simulink model "KUKA_KR10_R1100_1D"  (R2023b)
settings: Solver=ode15s  StartTime=0.0  StopTime=3  RelTol=1e-9  AbsTol=1e-9  EnableMultiTasking=on
values from neighbouring files (symbols this model uses):
  N = length(accelX)    [pds.m]
undefined symbols (not defined in the file or in its folder): X, Y, Z
libraries: nesl_utility x50, sm_lib x46
(part 1 of 2)
settings Model: Creator=beth0005  LastModifiedBy=Johannes
settings SolverCC: AutoScaleAbsTol=off  AlgebraicLoopSolver=TrustRegion
settings DataIOCC: LimitDataPoints=on  MaxDataPoints=10000
settings OptimizationCC: LifeSpan=inf
settings DebuggingCC: UnconnectedInputMsg=warning  UnconnectedOutputMsg=warning  UnconnectedLineMsg=warning  AllowSymbolicDim=off  SFUnexpectedBacktrackingDiag=warning  SFNoUnconditionalDefaultTransitionDiag=warning  SFExecutionAtInitializationDiag=none  ArithmeticOperatorsInVariantConditions=warning
settings ModelReferenceCC: EnableRefExpFcnMdlSchedulingChecks=on
settings SFSimCC: SimUseLocalCustomCode=off  CustomCodeUndefinedFunction=UseInterfaceOnly
settings RTWCC: RTWUseLocalCustomCode=off  DLArmComputeVersion=19.05
settings CodeAppCC: StateflowObjectComments=on
settings GRTTargetCC: TargetLangStandard=C89/C90 (ANSI)
settings ConfigComp: CovMetricSettings=dw  CovSaveCumulativeToWorkspaceVar=on  CovSaveSingleToWorkspaceVar=on  CovExternalEMLEnable=off  CovSFcnEnable=off
settings SimscapeCC: SimscapeLogType=all  SimscapeLogSimulationStatistics=on  SimscapeLogDataHistory=10000

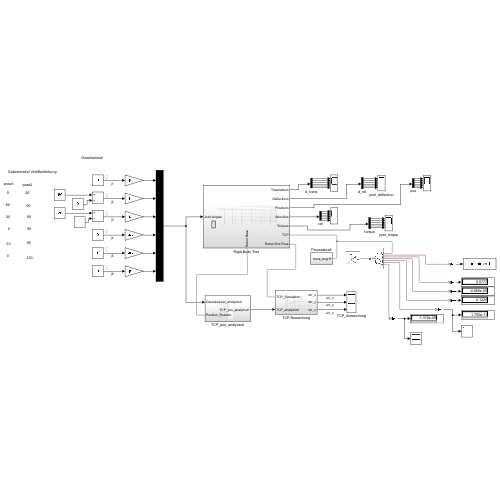
[thumbnail: Simulink's stored preview of the top-level diagram]
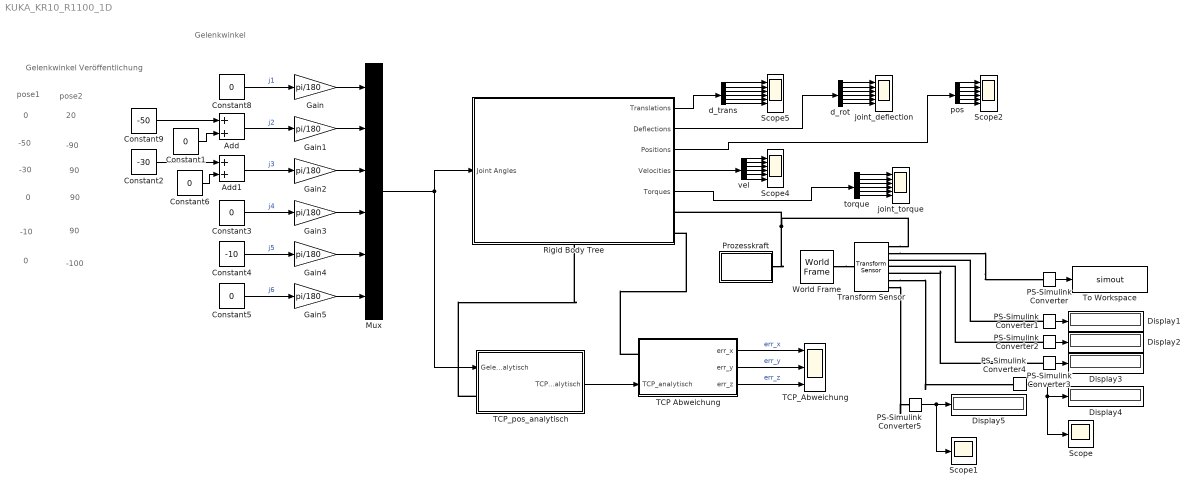
== system KUKA_KR10_R1100_1D ==
  note: -100
  note: pose2
  note: pose1
  note: 90
  note: 90
  note: 20
  note: 90
  note: -90
  note: Gelenkwinkel Veröffentlichung
  note: Gelenkwinkel
  note: 0
  note: -10
  note: 0
  note: 0
  note: -30
  note: -50
  Add : Sum
  Add1 : Sum
  Constant{1,3,5..6,8} (5 alike) : Constant  Value=0
  Constant2 : Constant  Value=-30
  Constant4 : Constant  Value=-10
  Constant9 : Constant  Value=-50
  Display{1..5} (5 alike) : Display
  Gain{,1..5} (6 alike) : Gain  Gain=pi/180
  Mux : Mux  Inputs=6
  PS-Simulink Converter{,1..5} (6 alike) : nesl_utility/PS-Simulink Converter  PhysicalDomain=network_engine_domain  SubClassName=ps_output  LeftPortType=input  RightPortType=output  PseudoPeriodic=off  Frequencies=[]  VectorFormat=inherit  Unit=inherit  AffineConversion=off
  Prozesskraft : Subsystem
  Rigid Body Tree : Subsystem
      settings: PortSchema="{\"entries\":[{\"content\":{\"sides\":[{\"content\":{\"connectorIds\":[\"In1\"]},\"type\":\"ConnectorPlacement.EquallySpacedRectSide\",\"uuid\":\"62483687-f9cb-4c30-88aa-fbca99035508\"},{\"content\":{\"connectorIds\":[\"Out1\",\"Out2\",\"Out3\",\"Out4\",\"Out5\",\"RConn1\",\"RConn2\"],\"side\":\"RIGHT\"},\"type\":\"ConnectorPlacement.EquallySpacedRectSide\",\"uuid\":\"72747b39-4529-4d6b-bc1f-f243ab09c1ee\"},{\"content\":{\"side\":\"TOP\"},\"type\":\"ConnectorPlacement.EquallySpacedRectSide\",\"uuid\":\"6a7c85b5-1fcd-47a7-a71b-25055be44f92\"},{\"content\":{\"connectorIds\":[\"RConn3\"],\"side\":\"BOTTOM\"},\"type\":\"ConnectorPlacement.EquallySpacedRectSide\",\"uuid\":\"78c07802-d245-487e-84d6-9da01077e918\"}]},\"type\":\"ConnectorPlacement.EquallySpacedConnector\",\"uuid\":\"7be79213-6e9f-4572-8e99-74e3fd1a1f63\"}],\"packageUris\":[\"http://schema.mathworks.com/mf0/Connector/R2020b\"],\"version\":\"1.0\"}"
  Scope : Scope
  Scope1 : Scope
  Scope2 : Scope  NumInputPorts=6
  Scope4 : Scope  NumInputPorts=6
  Scope5 : Scope  NumInputPorts=6
  TCP Abweichung : Subsystem
      settings: PortSchema="{\"entries\":[{\"content\":{\"sides\":[{\"content\":{\"connectorIds\":[\"LConn1\",\"In1\"]},\"type\":\"ConnectorPlacement.EquallySpacedRectSide\",\"uuid\":\"8fbb3f34-d7d1-4090-9281-a387436a6191\"},{\"content\":{\"connectorIds\":[\"Out1\",\"Out2\",\"Out3\"],\"side\":\"RIGHT\"},\"type\":\"ConnectorPlacement.EquallySpacedRectSide\",\"uuid\":\"2461bf91-e690-4063-84b2-ad7cc9454b37\"},{\"content\":{\"side\":\"TOP\"},\"type\":\"ConnectorPlacement.EquallySpacedRectSide\",\"uuid\":\"0fbb9cfb-49b2-42f2-b0a5-a9e967349aea\"}]},\"type\":\"ConnectorPlacement.EquallySpacedConnector\",\"uuid\":\"5e1e4f46-aaa2-4a76-a14e-db38171314b7\"}],\"packageUris\":[\"http://schema.mathworks.com/mf0/Connector/R2020b\"],\"version\":\"1.0\"}"
  TCP_Abweichung : Scope  NumInputPorts=3
  TCP_pos_analytisch : Subsystem
  To Workspace : ToWorkspace  VariableName=simout  SaveFormat=Structure  SampleTime=-1
  Transform Sensor : sm_lib/Frames and Transforms/Transform Sensor  MeasurementFrame=World  RotationSequence=XYX  SenseAngle=off  SenseAxis=off  SenseQ=off  SenseR=on  SenseRotationSequence=off  SenseOmegaX=off  SenseOmegaY=off  SenseOmegaZ=off  SenseOmega=off  SenseQDot=off  SenseRDot=off  SenseRotationSequenceDot=off  SenseAlphaX=off  SenseAlphaY=off  SenseAlphaZ=off  SenseAlpha=off  SenseQDDot=off  SenseRDDot=off  SenseX=on  SenseY=on  SenseZ=on  SenseXYZ=off  SenseRad=off  SenseAzim=off  SenseDist=off  SenseInc=off  SenseXDot=off  SenseYDot=off  SenseZDot=off  SenseXYZDot=on  SenseRadDot=off  SenseAzimDot=off  SenseDistDot=off  SenseIncDot=off  SenseXDDot=off  SenseYDDot=off  SenseZDDot=off  SenseXYZDDot=on  SenseRadDDot=off  SenseAzimDDot=off  SenseDistDDot=off  SenseIncDDot=off
  World Frame : sm_lib/Frames and Transforms/World Frame
  d_rot : Demux  Outputs=6
  d_trans : Demux  Outputs=6
  joint_deflection : Scope  NumInputPorts=6
  joint_torque : Scope  NumInputPorts=6
  pos : Demux  Outputs=6
  torque : Demux  Outputs=6
  vel : Demux  Outputs=6
  wires:
  Constant5/1 -> Gain5/1  "j6"
  Constant4/1 -> Gain4/1  "j5"
  Constant3/1 -> Gain3/1  "j4"
  d_rot/3 -> joint_deflection/3
  d_rot/6 -> joint_deflection/6
  d_rot/4 -> joint_deflection/4
  d_rot/5 -> joint_deflection/5
  d_rot/2 -> joint_deflection/2
  d_rot/1 -> joint_deflection/1
  pos/1 -> Scope2/1
  pos/2 -> Scope2/2
  pos/5 -> Scope2/5
  pos/4 -> Scope2/4
  pos/6 -> Scope2/6
  pos/3 -> Scope2/3
  torque/3 -> joint_torque/3
  torque/6 -> joint_torque/6
  torque/4 -> joint_torque/4
  torque/5 -> joint_torque/5
  torque/2 -> joint_torque/2
  torque/1 -> joint_torque/1
  vel/1 -> Scope4/1
  vel/2 -> Scope4/2
  vel/5 -> Scope4/5
  vel/4 -> Scope4/4
  vel/6 -> Scope4/6
  vel/3 -> Scope4/3
  d_trans/1 -> Scope5/1
  d_trans/2 -> Scope5/2
  d_trans/5 -> Scope5/5
  d_trans/4 -> Scope5/4
  d_trans/6 -> Scope5/6
  d_trans/3 -> Scope5/3
  TCP_pos_analytisch/1(TCP_pos_analytisch) -> TCP Abweichung/1(TCP_analytisch)
  TCP Abweichung/1(err_x) -> TCP_Abweichung/1  "err_x"
  TCP Abweichung/2(err_y) -> TCP_Abweichung/2  "err_y"
  TCP Abweichung/3(err_z) -> TCP_Abweichung/3  "err_z"
  Constant8/1 -> Gain/1  "j1"
  Gain/1 -> Mux/1
  Gain1/1 -> Mux/2
  Add/1 -> Gain1/1  "j2"
  Gain2/1 -> Mux/3
  Gain3/1 -> Mux/4
  Gain4/1 -> Mux/5
  Gain5/1 -> Mux/6
  Constant1/1 -> Add/2
  Constant6/1 -> Add1/2
  Add1/1 -> Gain2/1  "j3"
  PS-Simulink Converter1/1 -> Display1/1
  PS-Simulink Converter2/1 -> Display2/1
  PS-Simulink Converter3/1 -> Display3/1
  PS-Simulink Converter/1 -> To Workspace/1
  Constant9/1 -> Add/1
  Constant2/1 -> Add1/1
  PS-Simulink Converter4/1 -> Scope/1, Display4/1
  PS-Simulink Converter5/1 -> Scope1/1, Display5/1
  Mux/1 -> TCP_pos_analytisch/1(Gelenkwinkel_analytisch), Rigid Body Tree/1(Joint Angles)
  Rigid Body Tree/1(Translations) -> d_trans/1
  Rigid Body Tree/2(Deflections) -> d_rot/1
  Rigid Body Tree/3(Positions) -> pos/1
  Rigid Body Tree/4(Velocities) -> vel/1
  Rigid Body Tree/5(Torques) -> torque/1
  connections:
  World Frame/RConn1 -- Transform Sensor/LConn1
  Transform Sensor/RConn2 -- PS-Simulink Converter/LConn1
  PS-Simulink Converter1/LConn1 -- Transform Sensor/RConn3
  PS-Simulink Converter2/LConn1 -- Transform Sensor/RConn4
  PS-Simulink Converter3/LConn1 -- Transform Sensor/RConn5
  Transform Sensor/RConn6 -- PS-Simulink Converter4/LConn1
  Transform Sensor/RConn7 -- PS-Simulink Converter5/LConn1
  Prozesskraft/LConn1 -- Rigid Body Tree/RConn1 -- Transform Sensor/RConn1
  TCP_pos_analytisch/LConn1 -- Rigid Body Tree/RConn3
  TCP Abweichung/LConn1 -- Rigid Body Tree/RConn2

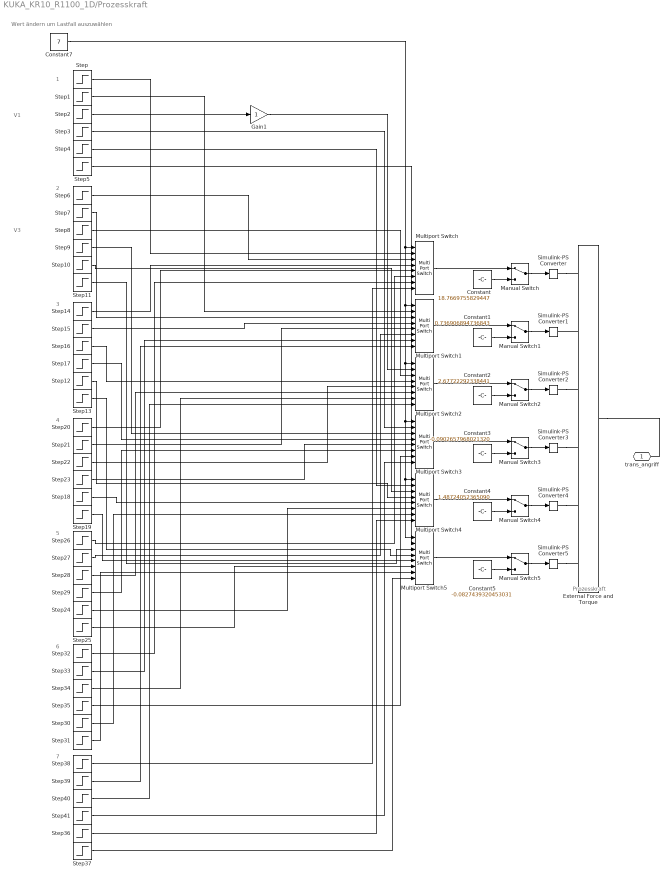
== system KUKA_KR10_R1100_1D/Prozesskraft ==
  note: Wert ändern um Lastfall auszuwählen
  note: V3
  note: V1
  note: Prozesskraft
  note: 1
  note: 2
  note: 3
  note: 4
  note: 5
  note: 6
  note: 7
  Constant : Constant  Value=18.7669755829447
  Constant1 : Constant  Value=0.736906894736843
  Constant2 : Constant  Value=2.67722292338441
  Constant3 : Constant  Value=-0.0902657968021320
  Constant4 : Constant  Value=1.48724052365090
  Constant5 : Constant  Value=-0.0827439320453031
  Constant7 : Constant  Value=7
  External Force and Torque : sm_lib/Forces and Torques/External Force and Torque  ForceResolutionFrame=AttachedFrame  EnableForceX=on  EnableForceY=on  EnableForceZ=on  EnableForce=off  TorqueResolutionFrame=AttachedFrame  EnableTorqueX=on  EnableTorqueY=on  EnableTorqueZ=on  EnableTorque=off
  Gain1 : Gain
  Manual Switch{,1..5} (6 alike) : ManualSwitch
  Multiport Switch{,1..5} (6 alike) : MultiPortSwitch  Inputs=7  SaturateOnIntegerOverflow=off  InputSameDT=off
  Simulink-PS Converter{,1..5} (6 alike) : nesl_utility/Simulink-PS Converter  PhysicalDomain=network_engine_domain  SubClassName=ps_input  LeftPortType=input  RightPortType=output  PseudoPeriodic=off  Frequencies=[]  NoiseDistribution=none  NoiseParameters=[]  Unit=1  AffineConversion=off  FilteringAndDerivatives=filter  SimscapeFilterOrder=2  InputFilterTimeConstant=0.001  UdotUserProvided=0
  Step : Step  Time=1.5  Before=10.45  After=0  SampleTime=0
  Step1 : Step  Time=1.5  Before=42.37  After=0  SampleTime=0
  Step10 : Step  Time=1.5  Before=0.27  After=0  SampleTime=0
  Step11 : Step  Time=1.5  Before=1.38  After=1.74  SampleTime=0
  Step12 : Step  Time=1.5  Before=0.47  After=0  SampleTime=0
  Step13 : Step  Time=1.5  Before=2.07  After=2.64  SampleTime=0
  Step14 : Step  Time=1.5  Before=8.44  After=0  SampleTime=0
  Step15 : Step  Time=1.5  Before=60.03  After=0  SampleTime=0
  Step16 : Step  Time=1.5  Before=-13.44  After=-47.67  SampleTime=0
  Step17 : Step  Time=1.5  Before=-0.03  After=0  SampleTime=0
  Step18 : Step  Time=1.5  Before=0.16  After=0  SampleTime=0
  Step19 : Step  Time=1.5  Before=2.36  After=3.01  SampleTime=0
  Step2 : Step  Time=1.5  Before=-7.82  After=-23.46  SampleTime=0
  Step20 : Step  Time=1.5  Before=6.32  After=0  SampleTime=0
  Step21 : Step  Time=1.5  Before=67.65  After=0  SampleTime=0
  Step22 : Step  Time=1.5  Before=-4.46  After=-25.52  SampleTime=0
  Step23 : Step  Time=1.5  Before=-0.02  After=0  SampleTime=0
  Step24 : Step  Time=1.5  Before=0.32  After=0  SampleTime=0
  Step25 : Step  Time=1.5  Before=3.54  After=4.54  SampleTime=0
  Step26 : Step  Time=1.5  Before=2.19  After=0  SampleTime=0
  Step27 : Step  Time=1.5  Before=102.5  After=0  SampleTime=0
  Step28 : Step  Time=1.5  Before=-9.11  After=-44.25  SampleTime=0
  Step29 : Step  Time=1.5  Before=-0.04  After=0  SampleTime=0
  Step3 : Step  Time=1.5  After=0  SampleTime=0
  Step30 : Step  Time=1.5  Before=0.3  After=0  SampleTime=0
  Step31 : Step  Time=1.5  Before=3.21  After=4.14  SampleTime=0
  Step32 : Step  Time=1.5  Before=1.98  After=0  SampleTime=0
  Step33 : Step  Time=1.5  Before=92.63  After=0  SampleTime=0
  Step34 : Step  Time=1.5  Before=-0.75  After=-22.78  SampleTime=0
  Step35 : Step  Time=1.5  Before=-0.03  After=0  SampleTime=0
  Step36 : Step  Time=1.5  Before=0.14  After=0  SampleTime=0
  Step37 : Step  Time=1.5  Before=4.83  After=6.22  SampleTime=0
  Step38 : Step  Time=1.5  Before=-5.57  After=0  SampleTime=0
  Step39 : Step  Time=1.5  Before=139.8  After=0  SampleTime=0
  Step4 : Step  Time=1.5  After=0  SampleTime=0
  Step40 : Step  Time=1.5  Before=-4.21  After=-40.32  SampleTime=0
  Step41 : Step  Time=1.5  Before=-0.05  After=0  SampleTime=0
  Step5 : Step  Time=1.5  Before=-1.462  After=-1.462  SampleTime=0
  Step6 : Step  Time=1.5  Before=9.11  After=0  SampleTime=0
  Step7 : Step  Time=1.5  Before=39.76  After=0  SampleTime=0
  Step8 : Step  Time=1.5  Before=-7.59  After=-28.04  SampleTime=0
  Step9 : Step  Time=1.5  Before=-0.02  After=0  SampleTime=0
  trans_angriff : PMIOPort  Side=Left
  wires:
  Constant7/1 -> Multiport Switch5/1, Multiport Switch4/1, Multiport Switch3/1, Multiport Switch2/1, Multiport Switch1/1, Multiport Switch/1
  Step/1 -> Multiport Switch/2
  Step1/1 -> Multiport Switch1/2
  Step2/1 -> Gain1/1
  Step3/1 -> Multiport Switch3/2
  Step4/1 -> Multiport Switch4/2
  Step5/1 -> Multiport Switch5/2
  Step6/1 -> Multiport Switch/3
  Step7/1 -> Multiport Switch1/3
  Step8/1 -> Multiport Switch2/3
  Step9/1 -> Multiport Switch3/3
  Step10/1 -> Multiport Switch4/3
  Step11/1 -> Multiport Switch5/3
  Step14/1 -> Multiport Switch/4
  Step15/1 -> Multiport Switch1/4
  Step16/1 -> Multiport Switch2/4
  Step17/1 -> Multiport Switch3/4
  Step12/1 -> Multiport Switch4/4
  Step13/1 -> Multiport Switch5/4
  Step20/1 -> Multiport Switch/5
  Step21/1 -> Multiport Switch1/5
  Step22/1 -> Multiport Switch2/5
  Step23/1 -> Multiport Switch3/5
  Step18/1 -> Multiport Switch4/5
  Step19/1 -> Multiport Switch5/5
  Step26/1 -> Multiport Switch/6
  Step27/1 -> Multiport Switch1/6
  Step28/1 -> Multiport Switch2/6
  Step29/1 -> Multiport Switch3/6
  Step24/1 -> Multiport Switch4/6
  Step25/1 -> Multiport Switch5/6
  Step32/1 -> Multiport Switch/7
  Step33/1 -> Multiport Switch1/7
  Step34/1 -> Multiport Switch2/7
  Step35/1 -> Multiport Switch3/7
  Step30/1 -> Multiport Switch4/7
  Step31/1 -> Multiport Switch5/7
  Step38/1 -> Multiport Switch/8
  Step39/1 -> Multiport Switch1/8
  Step40/1 -> Multiport Switch2/8
  Step41/1 -> Multiport Switch3/8
  Step36/1 -> Multiport Switch4/8
  Step37/1 -> Multiport Switch5/8
  Gain1/1 -> Multiport Switch2/2
  Multiport Switch/1 -> Manual Switch/1
  Manual Switch/1 -> Simulink-PS Converter/1
  Multiport Switch1/1 -> Manual Switch1/1
  Multiport Switch2/1 -> Manual Switch2/1
  Manual Switch2/1 -> Simulink-PS Converter2/1
  Manual Switch3/1 -> Simulink-PS Converter3/1
  Manual Switch4/1 -> Simulink-PS Converter4/1
  Manual Switch5/1 -> Simulink-PS Converter5/1
  Multiport Switch3/1 -> Manual Switch3/1
  Multiport Switch4/1 -> Manual Switch4/1
  Multiport Switch5/1 -> Manual Switch5/1
  Constant/1 -> Manual Switch/2
  Constant1/1 -> Manual Switch1/2
  Constant2/1 -> Manual Switch2/2
  Constant3/1 -> Manual Switch3/2
  Constant4/1 -> Manual Switch4/2
  Constant5/1 -> Manual Switch5/2
  Manual Switch1/1 -> Simulink-PS Converter1/1
  connections:
  Simulink-PS Converter4/RConn1 -- External Force and Torque/LConn5
  Simulink-PS Converter5/RConn1 -- External Force and Torque/LConn6
  Simulink-PS Converter3/RConn1 -- External Force and Torque/LConn4
  External Force and Torque/LConn2 -- Simulink-PS Converter1/RConn1
  Simulink-PS Converter2/RConn1 -- External Force and Torque/LConn3
  Simulink-PS Converter/RConn1 -- External Force and Torque/LConn1
  External Force and Torque/RConn1 -- trans_angriff/RConn1

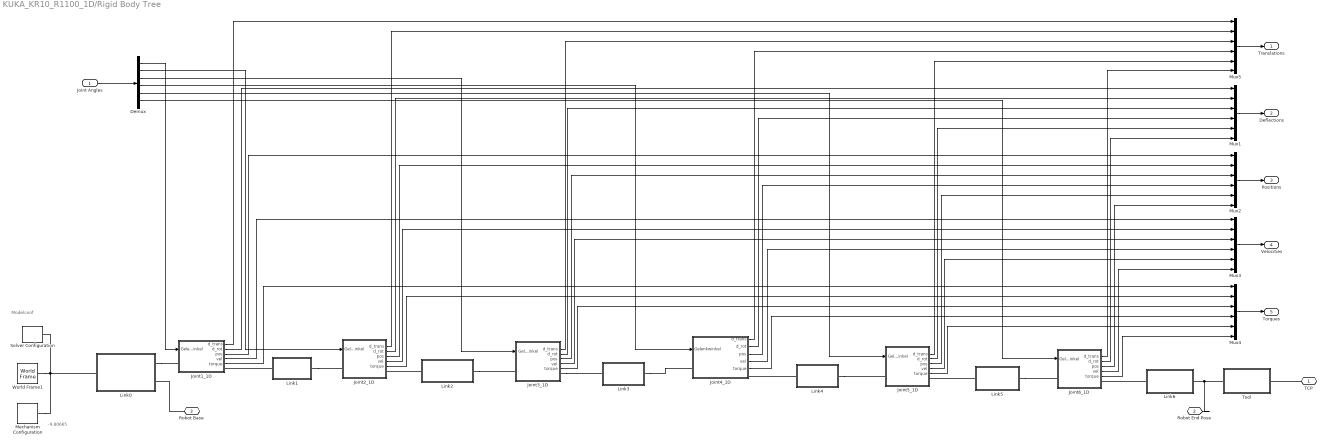
== system KUKA_KR10_R1100_1D/Rigid Body Tree ==
  note: Modelconf
  note: -9.80665
  Joint Angles : Inport
  Demux : Demux  Outputs=6
  Joint1_1D : Subsystem
  Joint2_1D : Subsystem
  Joint3_1D : Subsystem
  Joint4_1D : Subsystem
  Joint5_1D : Subsystem
  Joint6_1D : Subsystem
  Link0 : Subsystem
  Link1 : Subsystem
  Link2 : Subsystem
  Link3 : Subsystem
  Link4 : Subsystem
  Link5 : Subsystem
  Link6 : Subsystem
  Mechanism Configuration : sm_lib/Utilities/Mechanism Configuration  UniformGravity=Constant  GravityVector=[0 0 -9.80665]  GravityVectorUnits=m/s^2  LinearizationDelta=0.001  JointModeTransitionNonlinearIterations=2
  Mux{1..5} (5 alike) : Mux  Inputs=6
  Solver Configuration : nesl_utility/Solver Configuration  PhysicalDomain=network_engine_domain  SubClassName=solver  LeftPortType=input  RightPortType=generic  Tones=[]  Harmonics=[]  SimulateNoise=off  Profile=off  UseLocalSampling=off  EnableSwitchedLinearOptims=on  FrequencyDomain=off  UseCCode=off  RelTol=0.001  AbsTol=1e-06  MinStep=1e-09  ToWorkspace=off  RevertToSquareIcSolve=off  NumHomotopyIterations=100  PhasorMode=off  PhasorModeNumHarmonics=1  ConsistencySolver=NEWTON_FTOL  IndexReductionMethod=DerivativeReplacement  DoDC=off  ResidualTolerance=1e-09  ConsistencyTolSource=GLOBAL  ConsistencyAbsTol=0.001  ConsistencyRelTol=0.001  ConsistencyTolFactor=0.001  UseLocalSolver=off  LocalSolverChoice=NE_BACKWARD_EULER_ADVANCER  ResolveIndetEquations=on  FunctionEvalNumThread=1  LocalSolverSampleTime=0.001  DoFixedCost=off  MaxNonlinIter=3  MaxModeIter=2  ComputeImpulses=off  ImpulseIterations=2  LinearAlgebra=Sparse  LinearAlgebraNumThread=0  EquationFormulation=NE_TIME_EF  DelaysMemoryBudget=1024  AutomaticFiltering=on  FilteringTimeConstant=0.001  PartitionStorageMethod=AS_NEEDED  PartitionMemoryBudget=1024  PartitionMethod=FAST  MultibodyUseLocalSolver=off  MultibodyLocalSolverChoice=ODE1  MultibodyLocalSolverSampleTime=0.001
  Tool : Subsystem
  World Frame1 : sm_lib/Frames and Transforms/World Frame
  TCP : PMIOPort  Side=Right
  Robot End Pose : PMIOPort  Port=2  Side=Right
  Robot Base : PMIOPort  Port=3  Side=Right
  Translations : Outport
  Deflections : Outport  Port=2
  Positions : Outport  Port=3
  Velocities : Outport  Port=4
  Torques : Outport  Port=5
  wires:
  Joint2_1D/1(d_trans) -> Mux5/2
  Joint1_1D/4(vel) -> Mux3/1
  Joint2_1D/2(d_rot) -> Mux1/2
  Joint6_1D/5(torque) -> Mux4/6
  Joint Angles/1 -> Demux/1
  Joint3_1D/4(vel) -> Mux3/3
  Demux/2 -> Joint2_1D/1(Gelenkwinkel)
  Joint6_1D/1(d_trans) -> Mux5/6
  Joint6_1D/4(vel) -> Mux3/6
  Joint1_1D/5(torque) -> Mux4/1
  Joint2_1D/5(torque) -> Mux4/2
  Joint2_1D/4(vel) -> Mux3/2
  Joint4_1D/4(vel) -> Mux3/4
  Joint3_1D/3(pos) -> Mux2/3
  Joint2_1D/3(pos) -> Mux2/2
  Joint5_1D/4(vel) -> Mux3/5
  Joint5_1D/3(pos) -> Mux2/5
  Mux3/1 -> Velocities/1
  Joint6_1D/3(pos) -> Mux2/6
  Joint1_1D/2(d_rot) -> Mux1/1
  Joint4_1D/3(pos) -> Mux2/4
  Demux/4 -> Joint4_1D/1(Gelenkwinkel)
  Joint1_1D/3(pos) -> Mux2/1
  Joint6_1D/2(d_rot) -> Mux1/6
  Joint3_1D/5(torque) -> Mux4/3
  Joint4_1D/2(d_rot) -> Mux1/4
  Joint4_1D/1(d_trans) -> Mux5/4
  Joint1_1D/1(d_trans) -> Mux5/1
  Demux/6 -> Joint6_1D/1(Gelenkwinkel)
  Joint5_1D/1(d_trans) -> Mux5/5
  Joint3_1D/1(d_trans) -> Mux5/3
  Demux/5 -> Joint5_1D/1(Gelenkwinkel)
  Demux/3 -> Joint3_1D/1(Gelenkwinkel)
  Mux5/1 -> Translations/1
  Joint5_1D/2(d_rot) -> Mux1/5
  Joint5_1D/5(torque) -> Mux4/5
  Mux1/1 -> Deflections/1
  Joint3_1D/2(d_rot) -> Mux1/3
  Demux/1 -> Joint1_1D/1(Gelenkwinkel)
  Joint4_1D/5(torque) -> Mux4/4
  Mux2/1 -> Positions/1
  Mux4/1 -> Torques/1
  connections:
  Link2/LConn1 -- Joint2_1D/RConn1
  Link5/LConn1 -- Joint5_1D/RConn1
  Link5/RConn1 -- Joint6_1D/LConn1
  Link2/RConn1 -- Joint3_1D/LConn1
  Link1/LConn1 -- Joint1_1D/RConn1
  Link3/RConn1 -- Joint4_1D/LConn1
  World Frame1/RConn1 -- Mechanism Configuration/RConn1 -- Link0/LConn1 -- Solver Configuration/RConn1
  Joint3_1D/RConn1 -- Link3/LConn1
  Link1/RConn1 -- Joint2_1D/LConn1
  Tool/LConn1 -- Robot End Pose/RConn1 -- Link6/RConn1
  Link6/LConn1 -- Joint6_1D/RConn1
  TCP/RConn1 -- Tool/RConn1
  Link0/RConn1 -- Joint1_1D/LConn1
  Robot Base/RConn1 -- Link0/RConn2
  Link4/LConn1 -- Joint4_1D/RConn1
  Link4/RConn1 -- Joint5_1D/LConn1

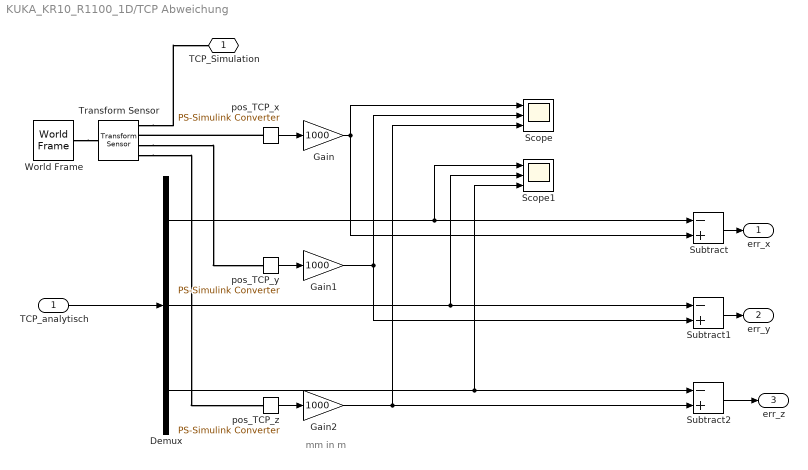
== system KUKA_KR10_R1100_1D/TCP Abweichung ==
  note: mm in m
  TCP_analytisch : Inport
  Demux : Demux  Outputs=3
  Gain : Gain  Gain=1000
  Gain1 : Gain  Gain=1000
  Gain2 : Gain  Gain=1000
  Scope : Scope  NumInputPorts=3
  Scope1 : Scope  NumInputPorts=3
  Subtract : Sum  Inputs=-+
  Subtract1 : Sum  Inputs=-+
  Subtract2 : Sum  Inputs=-+
  Transform Sensor : sm_lib/Frames and Transforms/Transform Sensor  MeasurementFrame=World  RotationSequence=XYX  SenseAngle=off  SenseAxis=off  SenseQ=off  SenseR=off  SenseRotationSequence=off  SenseOmegaX=off  SenseOmegaY=off  SenseOmegaZ=off  SenseOmega=off  SenseQDot=off  SenseRDot=off  SenseRotationSequenceDot=off  SenseAlphaX=off  SenseAlphaY=off  SenseAlphaZ=off  SenseAlpha=off  SenseQDDot=off  SenseRDDot=off  SenseX=on  SenseY=on  SenseZ=on  SenseXYZ=off  SenseRad=off  SenseAzim=off  SenseDist=off  SenseInc=off  SenseXDot=off  SenseYDot=off  SenseZDot=off  SenseXYZDot=off  SenseRadDot=off  SenseAzimDot=off  SenseDistDot=off  SenseIncDot=off  SenseXDDot=off  SenseYDDot=off  SenseZDDot=off  SenseXYZDDot=off  SenseRadDDot=off  SenseAzimDDot=off  SenseDistDDot=off  SenseIncDDot=off
  World Frame : sm_lib/Frames and Transforms/World Frame
  pos_TCP_x : nesl_utility/PS-Simulink Converter  PhysicalDomain=network_engine_domain  SubClassName=ps_output  LeftPortType=input  RightPortType=output  PseudoPeriodic=off  Frequencies=[]  VectorFormat=1-D array  Unit=inherit  AffineConversion=off
  pos_TCP_y : nesl_utility/PS-Simulink Converter  PhysicalDomain=network_engine_domain  SubClassName=ps_output  LeftPortType=input  RightPortType=output  PseudoPeriodic=off  Frequencies=[]  VectorFormat=1-D array  Unit=inherit  AffineConversion=off
  pos_TCP_z : nesl_utility/PS-Simulink Converter  PhysicalDomain=network_engine_domain  SubClassName=ps_output  LeftPortType=input  RightPortType=output  PseudoPeriodic=off  Frequencies=[]  VectorFormat=1-D array  Unit=inherit  AffineConversion=off
  TCP_Simulation : PMIOPort  Side=Left
  err_x : Outport
  err_y : Outport  Port=2
  err_z : Outport  Port=3
  wires:
  Demux/1 -> Scope1/1, Subtract/1
  Demux/2 -> Scope1/2, Subtract1/1
  Subtract1/1 -> err_y/1
  Subtract/1 -> err_x/1
  Subtract2/1 -> err_z/1
  TCP_analytisch/1 -> Demux/1
  Gain/1 -> Subtract/2, Scope/1
  Gain1/1 -> Scope/2, Subtract1/2
  pos_TCP_y/1 -> Gain1/1
  pos_TCP_z/1 -> Gain2/1
  Gain2/1 -> Scope/3, Subtract2/2
  pos_TCP_x/1 -> Gain/1
  Demux/3 -> Scope1/3, Subtract2/1
  connections:
  Transform Sensor/RConn3 -- pos_TCP_y/LConn1
  Transform Sensor/RConn4 -- pos_TCP_z/LConn1
  pos_TCP_x/LConn1 -- Transform Sensor/RConn2
  Transform Sensor/RConn1 -- TCP_Simulation/RConn1
  World Frame/RConn1 -- Transform Sensor/LConn1

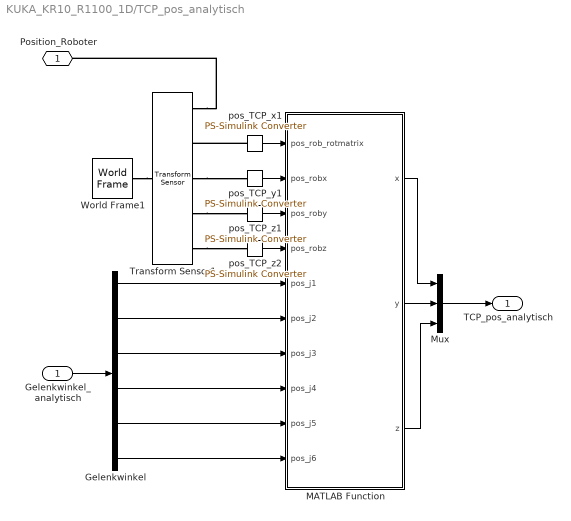
== system KUKA_KR10_R1100_1D/TCP_pos_analytisch ==
  Gelenkwinkel_analytisch : Inport
  Gelenkwinkel : Demux  Outputs=6
  MATLAB Function : MATLAB Function  TreatAsAtomicUnit=on
  Mux : Mux  Inputs=3
  Transform Sensor1 : sm_lib/Frames and Transforms/Transform Sensor  MeasurementFrame=World  RotationSequence=XYX  SenseAngle=off  SenseAxis=off  SenseQ=off  SenseR=on  SenseRotationSequence=off  SenseOmegaX=off  SenseOmegaY=off  SenseOmegaZ=off  SenseOmega=off  SenseQDot=off  SenseRDot=off  SenseRotationSequenceDot=off  SenseAlphaX=off  SenseAlphaY=off  SenseAlphaZ=off  SenseAlpha=off  SenseQDDot=off  SenseRDDot=off  SenseX=on  SenseY=on  SenseZ=on  SenseXYZ=off  SenseRad=off  SenseAzim=off  SenseDist=off  SenseInc=off  SenseXDot=off  SenseYDot=off  SenseZDot=off  SenseXYZDot=off  SenseRadDot=off  SenseAzimDot=off  SenseDistDot=off  SenseIncDot=off  SenseXDDot=off  SenseYDDot=off  SenseZDDot=off  SenseXYZDDot=off  SenseRadDDot=off  SenseAzimDDot=off  SenseDistDDot=off  SenseIncDDot=off
  World Frame1 : sm_lib/Frames and Transforms/World Frame
  pos_TCP_x1 : nesl_utility/PS-Simulink Converter  PhysicalDomain=network_engine_domain  SubClassName=ps_output  LeftPortType=input  RightPortType=output  PseudoPeriodic=off  Frequencies=[]  VectorFormat=1-D array  Unit=inherit  AffineConversion=off
  pos_TCP_y1 : nesl_utility/PS-Simulink Converter  PhysicalDomain=network_engine_domain  SubClassName=ps_output  LeftPortType=input  RightPortType=output  PseudoPeriodic=off  Frequencies=[]  VectorFormat=1-D array  Unit=inherit  AffineConversion=off
  pos_TCP_z1 : nesl_utility/PS-Simulink Converter  PhysicalDomain=network_engine_domain  SubClassName=ps_output  LeftPortType=input  RightPortType=output  PseudoPeriodic=off  Frequencies=[]  VectorFormat=1-D array  Unit=inherit  AffineConversion=off
  pos_TCP_z2 : nesl_utility/PS-Simulink Converter  PhysicalDomain=network_engine_domain  SubClassName=ps_output  LeftPortType=input  RightPortType=output  PseudoPeriodic=off  Frequencies=[]  VectorFormat=1-D array  Unit=inherit  AffineConversion=off
  Position_Roboter : PMIOPort  Side=Left
  TCP_pos_analytisch : Outport
  wires:
  Gelenkwinkel/3 -> MATLAB Function/7(pos_j3)
  Gelenkwinkel/6 -> MATLAB Function/10(pos_j6)
  Gelenkwinkel/1 -> MATLAB Function/5(pos_j1)
  pos_TCP_x1/1 -> MATLAB Function/1(pos_rob_rotmatrix)
  pos_TCP_y1/1 -> MATLAB Function/2(pos_robx)
  pos_TCP_z2/1 -> MATLAB Function/4(pos_robz)
  pos_TCP_z1/1 -> MATLAB Function/3(pos_roby)
  Gelenkwinkel_analytisch/1 -> Gelenkwinkel/1
  MATLAB Function/2(y) -> Mux/2
  Mux/1 -> TCP_pos_analytisch/1
  MATLAB Function/1(x) -> Mux/1
  MATLAB Function/3(z) -> Mux/3
  Gelenkwinkel/2 -> MATLAB Function/6(pos_j2)
  Gelenkwinkel/5 -> MATLAB Function/9(pos_j5)
  Gelenkwinkel/4 -> MATLAB Function/8(pos_j4)
  connections:
  Transform Sensor1/RConn3 -- pos_TCP_y1/LConn1
  World Frame1/RConn1 -- Transform Sensor1/LConn1
  Transform Sensor1/RConn5 -- pos_TCP_z2/LConn1
  pos_TCP_x1/LConn1 -- Transform Sensor1/RConn2
  Transform Sensor1/RConn4 -- pos_TCP_z1/LConn1
  Transform Sensor1/RConn1 -- Position_Roboter/RConn1

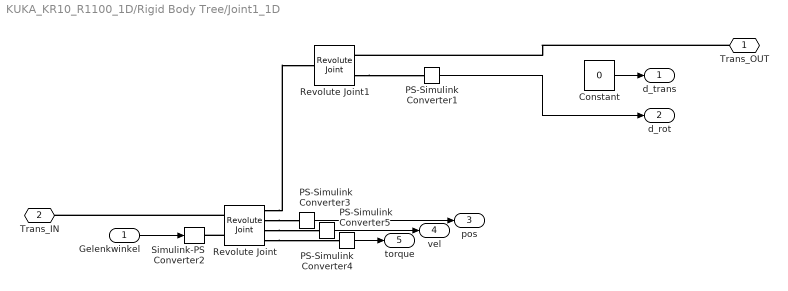
== system KUKA_KR10_R1100_1D/Rigid Body Tree/Joint1_1D ==
  Gelenkwinkel : Inport
  Constant : Constant  Value=0
  PS-Simulink Converter{1,3..5} (4 alike) : nesl_utility/PS-Simulink Converter  PhysicalDomain=network_engine_domain  SubClassName=ps_output  LeftPortType=input  RightPortType=output  PseudoPeriodic=off  Frequencies=[]  VectorFormat=1-D array  Unit=inherit  AffineConversion=off
  Revolute Joint : sm_lib/Joints/Revolute Joint  JointMode=Normal  SenseConstraintForce=off  SenseConstraintForceX=off  SenseConstraintForceY=off  SenseConstraintForceZ=off  SenseConstraintTorque=off  SenseConstraintTorqueX=off  SenseConstraintTorqueY=off  SenseConstraintTorqueZ=off  SenseTotalForce=off  SenseTotalForceX=off  SenseTotalForceY=off  SenseTotalForceZ=off  SenseTotalTorque=off  SenseTotalTorqueX=off  SenseTotalTorqueY=off  SenseTotalTorqueZ=off  CompositeWrenchDir=FollowerOnBase  CompositeWrenchFrame=BaseFrame  EquilibriumPosition=0  EquilibriumPositionUnits=deg  SpringStiffness=0  SpringStiffnessUnits=N*m/deg  DampingCoefficient=0  DampingCoefficientUnits=N*m/(deg/s)  TorqueActuationMode=ComputedTorque  MotionActuationMode=InputMotion  SensePosition=on  SenseVelocity=on  SenseAcceleration=off  SenseTorqueForce=on  SenseLowerLimitTorqueForce=off  SenseUpperLimitTorqueForce=off  LowerLimitSpecify=off  LowerLimitBound=-90  LowerLimitBoundUnits=deg  LowerLimitStiffness=1e4  LowerLimitStiffnessUnits=N*m/deg  LowerLimitDamping=10  LowerLimitDampingUnits=N*m/(deg/s)  LowerLimitTransitionRegionWidth=0.1  LowerLimitTransitionRegionWidthUnits=deg  UpperLimitSpecify=off  UpperLimitBound=90  UpperLimitBoundUnits=deg  UpperLimitStiffness=1e4  UpperLimitStiffnessUnits=N*m/deg  UpperLimitDamping=10  UpperLimitDampingUnits=N*m/(deg/s)  UpperLimitTransitionRegionWidth=0.1  UpperLimitTransitionRegionWidthUnits=deg  PositionTargetSpecify=off  PositionTargetPriority=High  PositionTargetValue=0  PositionTargetValueUnits=deg  VelocityTargetSpecify=off  VelocityTargetPriority=High  VelocityTargetValue=0  VelocityTargetValueUnits=deg/s
  Revolute Joint1 : sm_lib/Joints/Revolute Joint  JointMode=Normal  SenseConstraintForce=off  SenseConstraintForceX=off  SenseConstraintForceY=off  SenseConstraintForceZ=off  SenseConstraintTorque=off  SenseConstraintTorqueX=off  SenseConstraintTorqueY=off  SenseConstraintTorqueZ=off  SenseTotalForce=off  SenseTotalForceX=off  SenseTotalForceY=off  SenseTotalForceZ=off  SenseTotalTorque=off  SenseTotalTorqueX=off  SenseTotalTorqueY=off  SenseTotalTorqueZ=off  CompositeWrenchDir=FollowerOnBase  CompositeWrenchFrame=BaseFrame  EquilibriumPosition=0  EquilibriumPositionUnits=deg  SpringStiffness=j1_stiff  SpringStiffnessUnits=N*m/deg  DampingCoefficient=damp  DampingCoefficientUnits=N*m/(deg/s)  TorqueActuationMode=NoTorque  MotionActuationMode=ComputedMotion  SensePosition=on  SenseVelocity=off  SenseAcceleration=off  SenseTorqueForce=off  SenseLowerLimitTorqueForce=off  SenseUpperLimitTorqueForce=off  LowerLimitSpecify=off  LowerLimitBound=-90  LowerLimitBoundUnits=deg  LowerLimitStiffness=1e4  LowerLimitStiffnessUnits=N*m/deg  LowerLimitDamping=10  LowerLimitDampingUnits=N*m/(deg/s)  LowerLimitTransitionRegionWidth=0.1  LowerLimitTransitionRegionWidthUnits=deg  UpperLimitSpecify=off  UpperLimitBound=90  UpperLimitBoundUnits=deg  UpperLimitStiffness=1e4  UpperLimitStiffnessUnits=N*m/deg  UpperLimitDamping=10  UpperLimitDampingUnits=N*m/(deg/s)  UpperLimitTransitionRegionWidth=0.1  UpperLimitTransitionRegionWidthUnits=deg  PositionTargetSpecify=off  PositionTargetPriority=High  PositionTargetValue=0  PositionTargetValueUnits=deg  VelocityTargetSpecify=off  VelocityTargetPriority=High  VelocityTargetValue=0  VelocityTargetValueUnits=deg/s
  Simulink-PS Converter2 : nesl_utility/Simulink-PS Converter  PhysicalDomain=network_engine_domain  SubClassName=ps_input  LeftPortType=input  RightPortType=output  PseudoPeriodic=off  Frequencies=[]  NoiseDistribution=none  NoiseParameters=[]  Unit=1  AffineConversion=off  FilteringAndDerivatives=filter  SimscapeFilterOrder=2  InputFilterTimeConstant=0.001  UdotUserProvided=0
  Trans_OUT : PMIOPort  Side=Right
  Trans_IN : PMIOPort  Port=2  Side=Left
  d_trans : Outport
  d_rot : Outport  Port=2
  pos : Outport  Port=3
  vel : Outport  Port=4
  torque : Outport  Port=5
  wires:
  PS-Simulink Converter4/1 -> vel/1
  Gelenkwinkel/1 -> Simulink-PS Converter2/1
  PS-Simulink Converter5/1 -> torque/1
  PS-Simulink Converter3/1 -> pos/1
  PS-Simulink Converter1/1 -> d_rot/1
  Constant/1 -> d_trans/1
  connections:
  Revolute Joint/RConn4 -- PS-Simulink Converter5/LConn1
  Revolute Joint/RConn2 -- PS-Simulink Converter3/LConn1
  Revolute Joint/LConn2 -- Simulink-PS Converter2/RConn1
  Revolute Joint/RConn1 -- Revolute Joint1/LConn1
  Revolute Joint/RConn3 -- PS-Simulink Converter4/LConn1
  Revolute Joint/LConn1 -- Trans_IN/RConn1
  Trans_OUT/RConn1 -- Revolute Joint1/RConn1
  Revolute Joint1/RConn2 -- PS-Simulink Converter1/LConn1

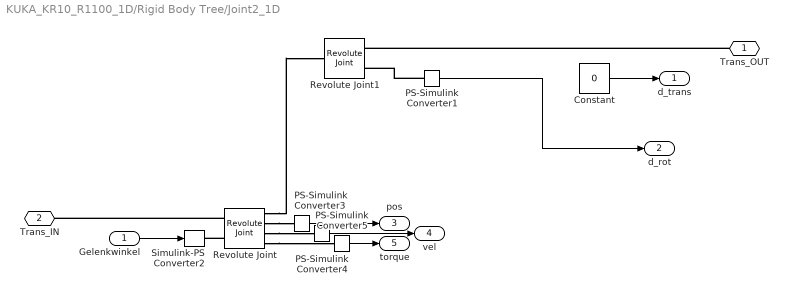
== system KUKA_KR10_R1100_1D/Rigid Body Tree/Joint2_1D ==
  Gelenkwinkel : Inport
  Constant : Constant  Value=0
  PS-Simulink Converter{1,3..5} (4 alike) : nesl_utility/PS-Simulink Converter  PhysicalDomain=network_engine_domain  SubClassName=ps_output  LeftPortType=input  RightPortType=output  PseudoPeriodic=off  Frequencies=[]  VectorFormat=1-D array  Unit=inherit  AffineConversion=off
  Revolute Joint : sm_lib/Joints/Revolute Joint  JointMode=Normal  SenseConstraintForce=off  SenseConstraintForceX=off  SenseConstraintForceY=off  SenseConstraintForceZ=off  SenseConstraintTorque=off  SenseConstraintTorqueX=off  SenseConstraintTorqueY=off  SenseConstraintTorqueZ=off  SenseTotalForce=off  SenseTotalForceX=off  SenseTotalForceY=off  SenseTotalForceZ=off  SenseTotalTorque=off  SenseTotalTorqueX=off  SenseTotalTorqueY=off  SenseTotalTorqueZ=off  CompositeWrenchDir=FollowerOnBase  CompositeWrenchFrame=BaseFrame  EquilibriumPosition=0  EquilibriumPositionUnits=deg  SpringStiffness=0  SpringStiffnessUnits=N*m/deg  DampingCoefficient=0  DampingCoefficientUnits=N*m/(deg/s)  TorqueActuationMode=ComputedTorque  MotionActuationMode=InputMotion  SensePosition=on  SenseVelocity=on  SenseAcceleration=off  SenseTorqueForce=on  SenseLowerLimitTorqueForce=off  SenseUpperLimitTorqueForce=off  LowerLimitSpecify=off  LowerLimitBound=-90  LowerLimitBoundUnits=deg  LowerLimitStiffness=1e4  LowerLimitStiffnessUnits=N*m/deg  LowerLimitDamping=10  LowerLimitDampingUnits=N*m/(deg/s)  LowerLimitTransitionRegionWidth=0.1  LowerLimitTransitionRegionWidthUnits=deg  UpperLimitSpecify=off  UpperLimitBound=90  UpperLimitBoundUnits=deg  UpperLimitStiffness=1e4  UpperLimitStiffnessUnits=N*m/deg  UpperLimitDamping=10  UpperLimitDampingUnits=N*m/(deg/s)  UpperLimitTransitionRegionWidth=0.1  UpperLimitTransitionRegionWidthUnits=deg  PositionTargetSpecify=off  PositionTargetPriority=High  PositionTargetValue=0  PositionTargetValueUnits=deg  VelocityTargetSpecify=off  VelocityTargetPriority=High  VelocityTargetValue=0  VelocityTargetValueUnits=deg/s
  Revolute Joint1 : sm_lib/Joints/Revolute Joint  JointMode=Normal  SenseConstraintForce=off  SenseConstraintForceX=off  SenseConstraintForceY=off  SenseConstraintForceZ=off  SenseConstraintTorque=off  SenseConstraintTorqueX=off  SenseConstraintTorqueY=off  SenseConstraintTorqueZ=off  SenseTotalForce=off  SenseTotalForceX=off  SenseTotalForceY=off  SenseTotalForceZ=off  SenseTotalTorque=off  SenseTotalTorqueX=off  SenseTotalTorqueY=off  SenseTotalTorqueZ=off  CompositeWrenchDir=FollowerOnBase  CompositeWrenchFrame=BaseFrame  EquilibriumPosition=0  EquilibriumPositionUnits=deg  SpringStiffness=j2_stiff  SpringStiffnessUnits=N*m/deg  DampingCoefficient=damp  DampingCoefficientUnits=N*m/(deg/s)  TorqueActuationMode=NoTorque  MotionActuationMode=ComputedMotion  SensePosition=on  SenseVelocity=off  SenseAcceleration=off  SenseTorqueForce=off  SenseLowerLimitTorqueForce=off  SenseUpperLimitTorqueForce=off  LowerLimitSpecify=off  LowerLimitBound=-90  LowerLimitBoundUnits=deg  LowerLimitStiffness=1e4  LowerLimitStiffnessUnits=N*m/deg  LowerLimitDamping=10  LowerLimitDampingUnits=N*m/(deg/s)  LowerLimitTransitionRegionWidth=0.1  LowerLimitTransitionRegionWidthUnits=deg  UpperLimitSpecify=off  UpperLimitBound=90  UpperLimitBoundUnits=deg  UpperLimitStiffness=1e4  UpperLimitStiffnessUnits=N*m/deg  UpperLimitDamping=10  UpperLimitDampingUnits=N*m/(deg/s)  UpperLimitTransitionRegionWidth=0.1  UpperLimitTransitionRegionWidthUnits=deg  PositionTargetSpecify=off  PositionTargetPriority=High  PositionTargetValue=0  PositionTargetValueUnits=deg  VelocityTargetSpecify=off  VelocityTargetPriority=High  VelocityTargetValue=0  VelocityTargetValueUnits=deg/s
  Simulink-PS Converter2 : nesl_utility/Simulink-PS Converter  PhysicalDomain=network_engine_domain  SubClassName=ps_input  LeftPortType=input  RightPortType=output  PseudoPeriodic=off  Frequencies=[]  NoiseDistribution=none  NoiseParameters=[]  Unit=1  AffineConversion=off  FilteringAndDerivatives=filter  SimscapeFilterOrder=2  InputFilterTimeConstant=0.001  UdotUserProvided=0
  Trans_OUT : PMIOPort  Side=Right
  Trans_IN : PMIOPort  Port=2  Side=Left
  d_trans : Outport
  d_rot : Outport  Port=2
  pos : Outport  Port=3
  vel : Outport  Port=4
  torque : Outport  Port=5
  wires:
  Gelenkwinkel/1 -> Simulink-PS Converter2/1
  PS-Simulink Converter1/1 -> d_rot/1
  PS-Simulink Converter5/1 -> torque/1
  PS-Simulink Converter3/1 -> pos/1
  PS-Simulink Converter4/1 -> vel/1
  Constant/1 -> d_trans/1
  connections:
  Trans_OUT/RConn1 -- Revolute Joint1/RConn1
  Revolute Joint/LConn1 -- Trans_IN/RConn1
  Revolute Joint/RConn1 -- Revolute Joint1/LConn1
  PS-Simulink Converter1/LConn1 -- Revolute Joint1/RConn2
  Revolute Joint/LConn2 -- Simulink-PS Converter2/RConn1
  Revolute Joint/RConn2 -- PS-Simulink Converter3/LConn1
  Revolute Joint/RConn4 -- PS-Simulink Converter5/LConn1
  Revolute Joint/RConn3 -- PS-Simulink Converter4/LConn1

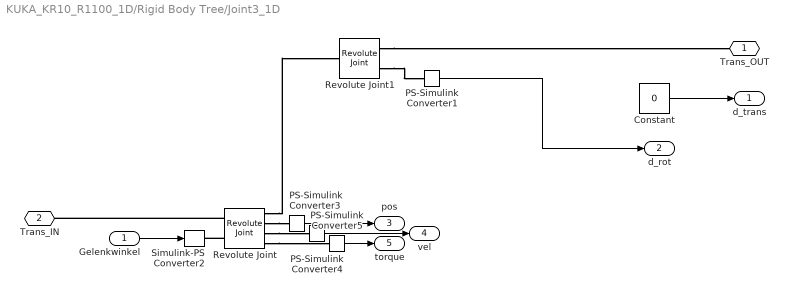
== system KUKA_KR10_R1100_1D/Rigid Body Tree/Joint3_1D ==
  Gelenkwinkel : Inport
  Constant : Constant  Value=0
  PS-Simulink Converter{1,3..5} (4 alike) : nesl_utility/PS-Simulink Converter  PhysicalDomain=network_engine_domain  SubClassName=ps_output  LeftPortType=input  RightPortType=output  PseudoPeriodic=off  Frequencies=[]  VectorFormat=1-D array  Unit=inherit  AffineConversion=off
  Revolute Joint : sm_lib/Joints/Revolute Joint  JointMode=Normal  SenseConstraintForce=off  SenseConstraintForceX=off  SenseConstraintForceY=off  SenseConstraintForceZ=off  SenseConstraintTorque=off  SenseConstraintTorqueX=off  SenseConstraintTorqueY=off  SenseConstraintTorqueZ=off  SenseTotalForce=off  SenseTotalForceX=off  SenseTotalForceY=off  SenseTotalForceZ=off  SenseTotalTorque=off  SenseTotalTorqueX=off  SenseTotalTorqueY=off  SenseTotalTorqueZ=off  CompositeWrenchDir=FollowerOnBase  CompositeWrenchFrame=BaseFrame  EquilibriumPosition=0  EquilibriumPositionUnits=deg  SpringStiffness=0  SpringStiffnessUnits=N*m/deg  DampingCoefficient=0  DampingCoefficientUnits=N*m/(deg/s)  TorqueActuationMode=ComputedTorque  MotionActuationMode=InputMotion  SensePosition=on  SenseVelocity=on  SenseAcceleration=off  SenseTorqueForce=on  SenseLowerLimitTorqueForce=off  SenseUpperLimitTorqueForce=off  LowerLimitSpecify=off  LowerLimitBound=-90  LowerLimitBoundUnits=deg  LowerLimitStiffness=1e4  LowerLimitStiffnessUnits=N*m/deg  LowerLimitDamping=10  LowerLimitDampingUnits=N*m/(deg/s)  LowerLimitTransitionRegionWidth=0.1  LowerLimitTransitionRegionWidthUnits=deg  UpperLimitSpecify=off  UpperLimitBound=90  UpperLimitBoundUnits=deg  UpperLimitStiffness=1e4  UpperLimitStiffnessUnits=N*m/deg  UpperLimitDamping=10  UpperLimitDampingUnits=N*m/(deg/s)  UpperLimitTransitionRegionWidth=0.1  UpperLimitTransitionRegionWidthUnits=deg  PositionTargetSpecify=off  PositionTargetPriority=High  PositionTargetValue=0  PositionTargetValueUnits=deg  VelocityTargetSpecify=off  VelocityTargetPriority=High  VelocityTargetValue=0  VelocityTargetValueUnits=deg/s
  Revolute Joint1 : sm_lib/Joints/Revolute Joint  JointMode=Normal  SenseConstraintForce=off  SenseConstraintForceX=off  SenseConstraintForceY=off  SenseConstraintForceZ=off  SenseConstraintTorque=off  SenseConstraintTorqueX=off  SenseConstraintTorqueY=off  SenseConstraintTorqueZ=off  SenseTotalForce=off  SenseTotalForceX=off  SenseTotalForceY=off  SenseTotalForceZ=off  SenseTotalTorque=off  SenseTotalTorqueX=off  SenseTotalTorqueY=off  SenseTotalTorqueZ=off  CompositeWrenchDir=FollowerOnBase  CompositeWrenchFrame=BaseFrame  EquilibriumPosition=0  EquilibriumPositionUnits=deg  SpringStiffness=j3_stiff  SpringStiffnessUnits=N*m/deg  DampingCoefficient=damp  DampingCoefficientUnits=N*m/(deg/s)  TorqueActuationMode=NoTorque  MotionActuationMode=ComputedMotion  SensePosition=on  SenseVelocity=off  SenseAcceleration=off  SenseTorqueForce=off  SenseLowerLimitTorqueForce=off  SenseUpperLimitTorqueForce=off  LowerLimitSpecify=off  LowerLimitBound=-90  LowerLimitBoundUnits=deg  LowerLimitStiffness=1e4  LowerLimitStiffnessUnits=N*m/deg  LowerLimitDamping=10  LowerLimitDampingUnits=N*m/(deg/s)  LowerLimitTransitionRegionWidth=0.1  LowerLimitTransitionRegionWidthUnits=deg  UpperLimitSpecify=off  UpperLimitBound=90  UpperLimitBoundUnits=deg  UpperLimitStiffness=1e4  UpperLimitStiffnessUnits=N*m/deg  UpperLimitDamping=10  UpperLimitDampingUnits=N*m/(deg/s)  UpperLimitTransitionRegionWidth=0.1  UpperLimitTransitionRegionWidthUnits=deg  PositionTargetSpecify=off  PositionTargetPriority=High  PositionTargetValue=0  PositionTargetValueUnits=deg  VelocityTargetSpecify=off  VelocityTargetPriority=High  VelocityTargetValue=0  VelocityTargetValueUnits=deg/s
  Simulink-PS Converter2 : nesl_utility/Simulink-PS Converter  PhysicalDomain=network_engine_domain  SubClassName=ps_input  LeftPortType=input  RightPortType=output  PseudoPeriodic=off  Frequencies=[]  NoiseDistribution=none  NoiseParameters=[]  Unit=1  AffineConversion=off  FilteringAndDerivatives=filter  SimscapeFilterOrder=2  InputFilterTimeConstant=0.001  UdotUserProvided=0
  Trans_OUT : PMIOPort  Side=Right
  Trans_IN : PMIOPort  Port=2  Side=Left
  d_trans : Outport
  d_rot : Outport  Port=2
  pos : Outport  Port=3
  vel : Outport  Port=4
  torque : Outport  Port=5
  wires:
  Gelenkwinkel/1 -> Simulink-PS Converter2/1
  PS-Simulink Converter1/1 -> d_rot/1
  PS-Simulink Converter5/1 -> torque/1
  PS-Simulink Converter3/1 -> pos/1
  PS-Simulink Converter4/1 -> vel/1
  Constant/1 -> d_trans/1
  connections:
  Revolute Joint/RConn2 -- PS-Simulink Converter3/LConn1
  Revolute Joint/LConn2 -- Simulink-PS Converter2/RConn1
  Revolute Joint1/RConn2 -- PS-Simulink Converter1/LConn1
  Revolute Joint/RConn1 -- Revolute Joint1/LConn1
  Revolute Joint/LConn1 -- Trans_IN/RConn1
  Revolute Joint1/RConn1 -- Trans_OUT/RConn1
  Revolute Joint/RConn4 -- PS-Simulink Converter5/LConn1
  Revolute Joint/RConn3 -- PS-Simulink Converter4/LConn1

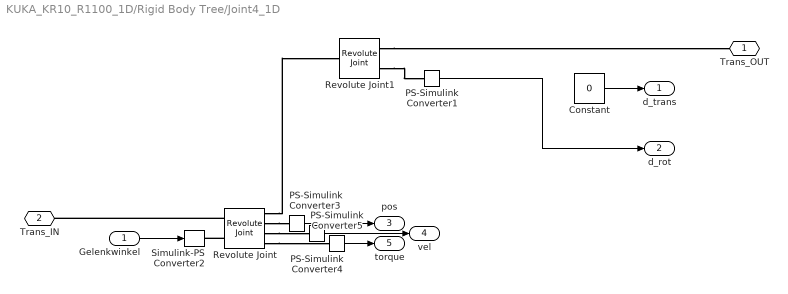
== system KUKA_KR10_R1100_1D/Rigid Body Tree/Joint4_1D ==
  Gelenkwinkel : Inport
  Constant : Constant  Value=0
  PS-Simulink Converter{1,3..5} (4 alike) : nesl_utility/PS-Simulink Converter  PhysicalDomain=network_engine_domain  SubClassName=ps_output  LeftPortType=input  RightPortType=output  PseudoPeriodic=off  Frequencies=[]  VectorFormat=1-D array  Unit=inherit  AffineConversion=off
  Revolute Joint : sm_lib/Joints/Revolute Joint  JointMode=Normal  SenseConstraintForce=off  SenseConstraintForceX=off  SenseConstraintForceY=off  SenseConstraintForceZ=off  SenseConstraintTorque=off  SenseConstraintTorqueX=off  SenseConstraintTorqueY=off  SenseConstraintTorqueZ=off  SenseTotalForce=off  SenseTotalForceX=off  SenseTotalForceY=off  SenseTotalForceZ=off  SenseTotalTorque=off  SenseTotalTorqueX=off  SenseTotalTorqueY=off  SenseTotalTorqueZ=off  CompositeWrenchDir=FollowerOnBase  CompositeWrenchFrame=BaseFrame  EquilibriumPosition=0  EquilibriumPositionUnits=deg  SpringStiffness=0  SpringStiffnessUnits=N*m/deg  DampingCoefficient=0  DampingCoefficientUnits=N*m/(deg/s)  TorqueActuationMode=ComputedTorque  MotionActuationMode=InputMotion  SensePosition=on  SenseVelocity=on  SenseAcceleration=off  SenseTorqueForce=on  SenseLowerLimitTorqueForce=off  SenseUpperLimitTorqueForce=off  LowerLimitSpecify=off  LowerLimitBound=-90  LowerLimitBoundUnits=deg  LowerLimitStiffness=1e4  LowerLimitStiffnessUnits=N*m/deg  LowerLimitDamping=10  LowerLimitDampingUnits=N*m/(deg/s)  LowerLimitTransitionRegionWidth=0.1  LowerLimitTransitionRegionWidthUnits=deg  UpperLimitSpecify=off  UpperLimitBound=90  UpperLimitBoundUnits=deg  UpperLimitStiffness=1e4  UpperLimitStiffnessUnits=N*m/deg  UpperLimitDamping=10  UpperLimitDampingUnits=N*m/(deg/s)  UpperLimitTransitionRegionWidth=0.1  UpperLimitTransitionRegionWidthUnits=deg  PositionTargetSpecify=off  PositionTargetPriority=High  PositionTargetValue=0  PositionTargetValueUnits=deg  VelocityTargetSpecify=off  VelocityTargetPriority=High  VelocityTargetValue=0  VelocityTargetValueUnits=deg/s
  Revolute Joint1 : sm_lib/Joints/Revolute Joint  JointMode=Normal  SenseConstraintForce=off  SenseConstraintForceX=off  SenseConstraintForceY=off  SenseConstraintForceZ=off  SenseConstraintTorque=off  SenseConstraintTorqueX=off  SenseConstraintTorqueY=off  SenseConstraintTorqueZ=off  SenseTotalForce=off  SenseTotalForceX=off  SenseTotalForceY=off  SenseTotalForceZ=off  SenseTotalTorque=off  SenseTotalTorqueX=off  SenseTotalTorqueY=off  SenseTotalTorqueZ=off  CompositeWrenchDir=FollowerOnBase  CompositeWrenchFrame=BaseFrame  EquilibriumPosition=0  EquilibriumPositionUnits=deg  SpringStiffness=j4_stiff  SpringStiffnessUnits=N*m/deg  DampingCoefficient=damp  DampingCoefficientUnits=N*m/(deg/s)  TorqueActuationMode=NoTorque  MotionActuationMode=ComputedMotion  SensePosition=on  SenseVelocity=off  SenseAcceleration=off  SenseTorqueForce=off  SenseLowerLimitTorqueForce=off  SenseUpperLimitTorqueForce=off  LowerLimitSpecify=off  LowerLimitBound=-90  LowerLimitBoundUnits=deg  LowerLimitStiffness=1e4  LowerLimitStiffnessUnits=N*m/deg  LowerLimitDamping=10  LowerLimitDampingUnits=N*m/(deg/s)  LowerLimitTransitionRegionWidth=0.1  LowerLimitTransitionRegionWidthUnits=deg  UpperLimitSpecify=off  UpperLimitBound=90  UpperLimitBoundUnits=deg  UpperLimitStiffness=1e4  UpperLimitStiffnessUnits=N*m/deg  UpperLimitDamping=10  UpperLimitDampingUnits=N*m/(deg/s)  UpperLimitTransitionRegionWidth=0.1  UpperLimitTransitionRegionWidthUnits=deg  PositionTargetSpecify=off  PositionTargetPriority=High  PositionTargetValue=0  PositionTargetValueUnits=deg  VelocityTargetSpecify=off  VelocityTargetPriority=High  VelocityTargetValue=0  VelocityTargetValueUnits=deg/s
  Simulink-PS Converter2 : nesl_utility/Simulink-PS Converter  PhysicalDomain=network_engine_domain  SubClassName=ps_input  LeftPortType=input  RightPortType=output  PseudoPeriodic=off  Frequencies=[]  NoiseDistribution=none  NoiseParameters=[]  Unit=1  AffineConversion=off  FilteringAndDerivatives=filter  SimscapeFilterOrder=2  InputFilterTimeConstant=0.001  UdotUserProvided=0
  Trans_OUT : PMIOPort  Side=Right
  Trans_IN : PMIOPort  Port=2  Side=Left
  d_trans : Outport
  d_rot : Outport  Port=2
  pos : Outport  Port=3
  vel : Outport  Port=4
  torque : Outport  Port=5
  wires:
  Gelenkwinkel/1 -> Simulink-PS Converter2/1
  PS-Simulink Converter1/1 -> d_rot/1
  PS-Simulink Converter5/1 -> torque/1
  PS-Simulink Converter3/1 -> pos/1
  PS-Simulink Converter4/1 -> vel/1
  Constant/1 -> d_trans/1
  connections:
  Revolute Joint1/RConn1 -- Trans_OUT/RConn1
  Revolute Joint/LConn1 -- Trans_IN/RConn1
  Revolute Joint/RConn1 -- Revolute Joint1/LConn1
  Revolute Joint1/RConn2 -- PS-Simulink Converter1/LConn1
  Revolute Joint/LConn2 -- Simulink-PS Converter2/RConn1
  Revolute Joint/RConn2 -- PS-Simulink Converter3/LConn1
  Revolute Joint/RConn4 -- PS-Simulink Converter5/LConn1
  Revolute Joint/RConn3 -- PS-Simulink Converter4/LConn1

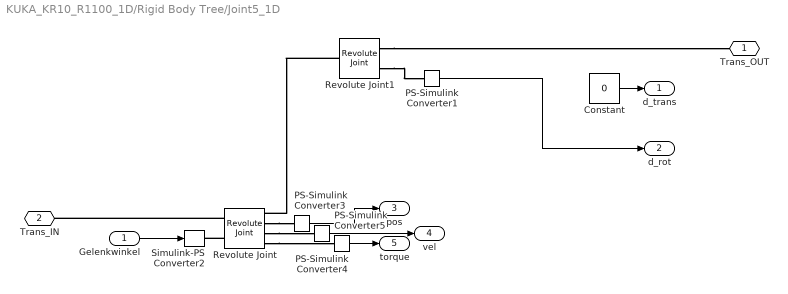
== system KUKA_KR10_R1100_1D/Rigid Body Tree/Joint5_1D ==
  Gelenkwinkel : Inport
  Constant : Constant  Value=0
  PS-Simulink Converter{1,3..5} (4 alike) : nesl_utility/PS-Simulink Converter  PhysicalDomain=network_engine_domain  SubClassName=ps_output  LeftPortType=input  RightPortType=output  PseudoPeriodic=off  Frequencies=[]  VectorFormat=1-D array  Unit=inherit  AffineConversion=off
  Revolute Joint : sm_lib/Joints/Revolute Joint  JointMode=Normal  SenseConstraintForce=off  SenseConstraintForceX=off  SenseConstraintForceY=off  SenseConstraintForceZ=off  SenseConstraintTorque=off  SenseConstraintTorqueX=off  SenseConstraintTorqueY=off  SenseConstraintTorqueZ=off  SenseTotalForce=off  SenseTotalForceX=off  SenseTotalForceY=off  SenseTotalForceZ=off  SenseTotalTorque=off  SenseTotalTorqueX=off  SenseTotalTorqueY=off  SenseTotalTorqueZ=off  CompositeWrenchDir=FollowerOnBase  CompositeWrenchFrame=BaseFrame  EquilibriumPosition=0  EquilibriumPositionUnits=deg  SpringStiffness=0  SpringStiffnessUnits=N*m/deg  DampingCoefficient=0  DampingCoefficientUnits=N*m/(deg/s)  TorqueActuationMode=ComputedTorque  MotionActuationMode=InputMotion  SensePosition=on  SenseVelocity=on  SenseAcceleration=off  SenseTorqueForce=on  SenseLowerLimitTorqueForce=off  SenseUpperLimitTorqueForce=off  LowerLimitSpecify=off  LowerLimitBound=-90  LowerLimitBoundUnits=deg  LowerLimitStiffness=1e4  LowerLimitStiffnessUnits=N*m/deg  LowerLimitDamping=10  LowerLimitDampingUnits=N*m/(deg/s)  LowerLimitTransitionRegionWidth=0.1  LowerLimitTransitionRegionWidthUnits=deg  UpperLimitSpecify=off  UpperLimitBound=90  UpperLimitBoundUnits=deg  UpperLimitStiffness=1e4  UpperLimitStiffnessUnits=N*m/deg  UpperLimitDamping=10  UpperLimitDampingUnits=N*m/(deg/s)  UpperLimitTransitionRegionWidth=0.1  UpperLimitTransitionRegionWidthUnits=deg  PositionTargetSpecify=off  PositionTargetPriority=High  PositionTargetValue=0  PositionTargetValueUnits=deg  VelocityTargetSpecify=off  VelocityTargetPriority=High  VelocityTargetValue=0  VelocityTargetValueUnits=deg/s
  Revolute Joint1 : sm_lib/Joints/Revolute Joint  JointMode=Normal  SenseConstraintForce=off  SenseConstraintForceX=off  SenseConstraintForceY=off  SenseConstraintForceZ=off  SenseConstraintTorque=off  SenseConstraintTorqueX=off  SenseConstraintTorqueY=off  SenseConstraintTorqueZ=off  SenseTotalForce=off  SenseTotalForceX=off  SenseTotalForceY=off  SenseTotalForceZ=off  SenseTotalTorque=off  SenseTotalTorqueX=off  SenseTotalTorqueY=off  SenseTotalTorqueZ=off  CompositeWrenchDir=FollowerOnBase  CompositeWrenchFrame=BaseFrame  EquilibriumPosition=0  EquilibriumPositionUnits=deg  SpringStiffness=j5_stiff  SpringStiffnessUnits=N*m/deg  DampingCoefficient=damp  DampingCoefficientUnits=N*m/(deg/s)  TorqueActuationMode=NoTorque  MotionActuationMode=ComputedMotion  SensePosition=on  SenseVelocity=off  SenseAcceleration=off  SenseTorqueForce=off  SenseLowerLimitTorqueForce=off  SenseUpperLimitTorqueForce=off  LowerLimitSpecify=off  LowerLimitBound=-90  LowerLimitBoundUnits=deg  LowerLimitStiffness=1e4  LowerLimitStiffnessUnits=N*m/deg  LowerLimitDamping=10  LowerLimitDampingUnits=N*m/(deg/s)  LowerLimitTransitionRegionWidth=0.1  LowerLimitTransitionRegionWidthUnits=deg  UpperLimitSpecify=off  UpperLimitBound=90  UpperLimitBoundUnits=deg  UpperLimitStiffness=1e4  UpperLimitStiffnessUnits=N*m/deg  UpperLimitDamping=10  UpperLimitDampingUnits=N*m/(deg/s)  UpperLimitTransitionRegionWidth=0.1  UpperLimitTransitionRegionWidthUnits=deg  PositionTargetSpecify=off  PositionTargetPriority=High  PositionTargetValue=0  PositionTargetValueUnits=deg  VelocityTargetSpecify=off  VelocityTargetPriority=High  VelocityTargetValue=0  VelocityTargetValueUnits=deg/s
  Simulink-PS Converter2 : nesl_utility/Simulink-PS Converter  PhysicalDomain=network_engine_domain  SubClassName=ps_input  LeftPortType=input  RightPortType=output  PseudoPeriodic=off  Frequencies=[]  NoiseDistribution=none  NoiseParameters=[]  Unit=1  AffineConversion=off  FilteringAndDerivatives=filter  SimscapeFilterOrder=2  InputFilterTimeConstant=0.001  UdotUserProvided=0
  Trans_OUT : PMIOPort  Side=Right
  Trans_IN : PMIOPort  Port=2  Side=Left
  d_trans : Outport
  d_rot : Outport  Port=2
  pos : Outport  Port=3
  vel : Outport  Port=4
  torque : Outport  Port=5
  wires:
  Gelenkwinkel/1 -> Simulink-PS Converter2/1
  PS-Simulink Converter1/1 -> d_rot/1
  PS-Simulink Converter5/1 -> torque/1
  PS-Simulink Converter3/1 -> pos/1
  PS-Simulink Converter4/1 -> vel/1
  Constant/1 -> d_trans/1
  connections:
  Revolute Joint/RConn2 -- PS-Simulink Converter3/LConn1
  Revolute Joint/LConn2 -- Simulink-PS Converter2/RConn1
  Revolute Joint1/RConn2 -- PS-Simulink Converter1/LConn1
  Revolute Joint1/LConn1 -- Revolute Joint/RConn1
  Revolute Joint/LConn1 -- Trans_IN/RConn1
  Revolute Joint1/RConn1 -- Trans_OUT/RConn1
  Revolute Joint/RConn4 -- PS-Simulink Converter5/LConn1
  Revolute Joint/RConn3 -- PS-Simulink Converter4/LConn1
